simulink model "MPPT_solar_sim"  (R2019b)
settings: Solver=VariableStepAuto  StartTime=0.0  StopTime=10  RelTol=1e-3
undefined symbols (not defined in the file or in its folder): sigbuilder_block
libraries: powerlib x10, re_lib x1, powerlib_meascontrol x1
settings Model: Creator=root  LastModifiedBy=root

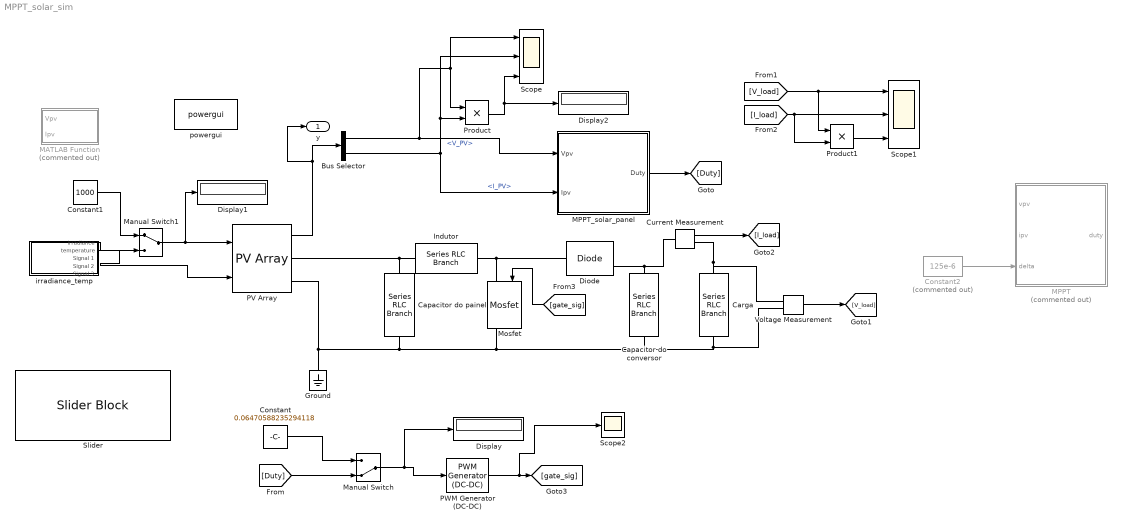
== system MPPT_solar_sim ==
  Bus Selector : BusSelector  OutputSignals=V_PV,I_PV
  Capacitor do conversor : powerlib/Elements/Series RLC Branch  LConnTagsString=__new0  RConnTagsString=__new0  BranchType=C  Resistance=1e-4  Inductance=1e-3  SetiL0=off  InitialCurrent=0  Capacitance=500e-6  Setx0=off  InitialVoltage=0  Measurements=None
      settings: SourceProductName=Simscape Electrical
  Capacitor do painel : powerlib/Elements/Series RLC Branch  LConnTagsString=__new0  RConnTagsString=__new0  BranchType=C  Resistance=1e-4  Inductance=1e-3  SetiL0=off  InitialCurrent=0  Capacitance=100e-6  Setx0=off  InitialVoltage=0  Measurements=None
      settings: SourceProductName=Simscape Electrical
  "Carga " : powerlib/Elements/Series RLC Branch  LConnTagsString=__new0  RConnTagsString=__new0  BranchType=R  Resistance=10  Inductance=1e-3  SetiL0=off  InitialCurrent=0  Capacitance=20e-6  Setx0=off  InitialVoltage=0  Measurements=None
      settings: SourceProductName=Simscape Electrical
  Constant : Constant  Value=0.06470588235294118
  Constant1 : Constant  Value=1000
  Constant2 : Constant  Commented=on  Value=125e-6
  Current Measurement : powerlib/Measurements/Current Measurement  PhasorSimulation=off  OutputType=Complex  PSBequivalent=0
      settings: SourceProductName=Simscape Electrical
  Diode : powerlib/Power Electronics/Diode  Ron=0.001  Lon=0  Vf=0.8  IC=0  UseSnubber=0  Rs=500  Cs=250e-9  Measurements=on
      settings: SourceProductName=Simscape Electrical
  Display : Display
  Display1 : Display
  Display2 : Display
  Ground : powerlib/Elements/Ground  LConnTagsString=a
      settings: SourceProductName=Simscape Electrical
  Indutor : powerlib/Elements/Series RLC Branch  LConnTagsString=__new0  RConnTagsString=__new0  BranchType=L  Resistance=1e-4  Inductance=235e-6  SetiL0=off  InitialCurrent=0  Capacitance=100e-6  Setx0=off  InitialVoltage=0  Measurements=None
      settings: SourceProductName=Simscape Electrical
  MATLAB Function : MATLAB Function  Commented=on  TreatAsAtomicUnit=on
  MPPT : MATLAB Function  Commented=on  TreatAsAtomicUnit=on
  "MPPT_solar_panel " : MATLAB Function  TreatAsAtomicUnit=on
  Manual Switch : ManualSwitch  CurrentSetting=0
  Manual Switch1 : ManualSwitch
  Mosfet : powerlib/Power Electronics/Mosfet  Ron=0.1  Lon=0  Rd=0.01  Vfd=0  IC=0  Rs=1e5  Cs=inf  Measurements=on
      settings: SourceProductName=Simscape Electrical
  PV Array : re_lib/Solar/PV Array  Npar=1  Nser=1  PlotType=one module @ 25 deg.C & specified irradiances  S_vec="[ 1000  800  600 400 200]"  Temp_C_vec="[ 45 25  ]"  ModuleName=User-defined  PlotWhenSelected=off  Pm=400.488  Ncell=60  Voc=48.70  Isc=10.79  Vm=40.70  Im=9.84  beta_Voc_pc=-0.289  alpha_Isc_pc=0.051  beta_Voc=-0.14074  alpha_Isc=0.0055029  IL=10.8217  I0=2.2788e-11  nI=1.1776  Rsh=79.7466  Rs=0.23394  BAL=on  Tc=1e-6  Tfilter=1e-3
      settings: SourceProductName=Simscape Electrical
  PWM Generator (DC-DC) : powerlib_meascontrol/Pulse & Signal Generators/PWM Generator (DC-DC)  Fsw=30e3  Ts=0
      settings: SourceProductName=Simscape Electrical
  Product : Product
  Product1 : Product
  Scope : Scope  NumInputPorts=3
  Scope1 : Scope  NumInputPorts=3
  Scope2 : Scope
  Slider : SliderBlock  ScaleMax=1
  Voltage Measurement : powerlib/Measurements/Voltage Measurement  PhasorSimulation=off  OutputType=Complex  PSBequivalent=0
      settings: SourceProductName=Simscape Electrical
  irradiance_temp : Subsystem  Tag=STV Subsys  LoadFcn=sigbuilder_block('load');  StartFcn=sigbuilder_block('start');  StopFcn=sigbuilder_block('stop');  ClipboardFcn=sigbuilder_block('clipboard');  mask(Sigbuilder block){tuvar=[0:10]}
      mask help: Simulink:masks:SigbuilderBlock_MD
      mask init:
      | if ~strcmp(get_param(bdroot(gcbh),'SimulationStatus'),'stopped') tuvar = sigbuilder_block('maskInit'); end
      settings: CopyFcn=sigbuilder_block('copy');  DeleteFcn=sigbuilder_block('delete');  ModelCloseFcn=sigbuilder_block('modelClose');  PreSaveFcn=sigbuilder_block('preSave');  PauseFcn=sigbuilder_block('pause');  ContinueFcn=sigbuilder_block('continue');  NameChangeFcn=sigbuilder_block('namechange');  OpenFcn=sigbuilder_block('open',[0 0 1868.11 814.378 ]);  CloseFcn=sigbuilder_block('close');
      mask Display: plot(0, 0, 100, 100,[2, 2, 32, 32, 2], [68, 8, 8, 68, 68],[32, 2], [38, 38], [32, 19, 2],[53, 60, 44], [32, 17, 17, 2],[16, 16, 31, 31]);txt = getActiveGroup(gcbh);text(2, 100, txt,'verticalAlignment', 'top');
  powergui : powerlib/powergui  Priority=1  SimulationMode=Discrete  SampleTime=1e-6  frequency=60  Iterations=50  frequencyindice=0  Pbase=100e6  ErrMax=1e-4  UnitsV=kV  UnitsW=MW  buscounter=0  FunctionMessages=off  echomessages=off  EnableUseOfTLC=off  CurrentSourceSwitches=off  DisableSnubberDevices=off  DisableRonSwitches=off  DisableVfSwitches=off  DisplayEquations=off  AutomaticDiscreteSolvers=off  SolverType=Tustin/Backward Euler (TBE)  Interpol=off  ExternalGateDelay=off  methode=off  Ts=100  x0status=blocks  SPID=on  SwTol=0  HookPort=off  NonlinearTolerance=1e-4  nMaxIteration=100  ContinueOnMaxIteration=off  RestoreLinks=warning  ResistiveCurrentMeasurement=off  Frange=[0:2:500]  Ylog=off  Xlog=on  ShowGrid=off  save=off  variable=ZData  structure=0  ZoomFFT=off  StartTime=0.0  cycles=1  DisplayStyle=1  fundamental=60  FreqAxis=off  MaxFrequency=1000  frequencyindicesteady=1  RmsSteady=1  display=off
      settings: SourceProductName=Simscape Electrical
  " y" : Outport
  wires:
  Bus Selector/1 -> "MPPT_solar_panel "/1(Vpv), Product/1, Scope/1  "<V_PV>"
  Bus Selector/2 -> "MPPT_solar_panel "/2(Ipv), Scope/2, Product/2  "<I_PV>"
  PV Array/1 -> Bus Selector/1, " y"/1
  irradiance_temp/2(temperature) -> PV Array/2
  Voltage Measurement/1 -> [V_load]
  Current Measurement/1 -> [I_load]
  [V_load] -> Product1/1, Scope1/1
  [I_load] -> Scope1/2, Product1/2
  PWM Generator (DC-DC)/1 -> Scope2/1, [gate_sig]
  Product/1 -> Display2/1, Scope/3
  [Duty] -> Manual Switch/2
  Manual Switch/1 -> Display/1, PWM Generator (DC-DC)/1
  Constant/1 -> Manual Switch/1
  Product1/1 -> Scope1/3
  irradiance_temp/1(irradiance) -> Manual Switch1/2
  Manual Switch1/1 -> Display1/1, PV Array/1
  Constant1/1 -> Manual Switch1/1
  [gate_sig] -> Mosfet/1
  Constant2/1 -> MPPT/3(delta)
  "MPPT_solar_panel "/1(Duty) -> [Duty]
  connections:
  PV Array/RConn2 -- Mosfet/RConn1 -- Voltage Measurement/LConn2 -- "Carga "/RConn1 -- Capacitor do conversor/RConn1 -- Capacitor do painel/RConn1 -- Ground/LConn1
  "Carga "/LConn1 -- Voltage Measurement/LConn1 -- Current Measurement/RConn1
  Current Measurement/LConn1 -- Diode/RConn1 -- Capacitor do conversor/LConn1
  Capacitor do painel/LConn1 -- PV Array/RConn1 -- Indutor/RConn1
  Mosfet/LConn1 -- Diode/LConn1 -- Indutor/LConn1

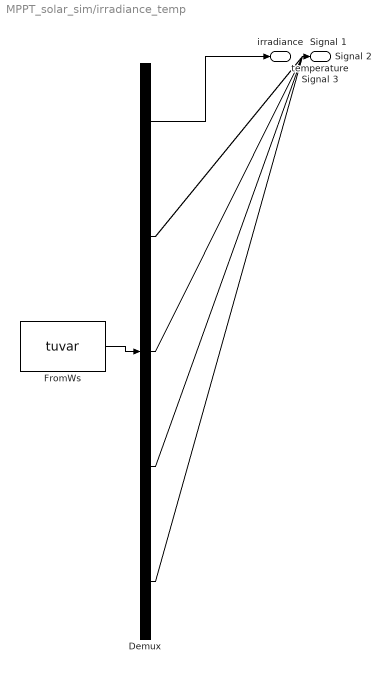
== system MPPT_solar_sim/irradiance_temp ==
  Demux : Demux  Tag=STV Demux  Outputs=5
  FromWs : FromWorkspace  Tag=STV FromWs  VariableName=tuvar  SampleTime=0
      SigBuilderData=|
      | common.afterFinalStr = 'Extrapolate'
      | common.sampleTime = 0
      | dataSet.timeRange = [0 10]
      | dataSet.name = 'Group 1'
      | sbobj.Groups.Name = 'Group 1'
      | sbobj.Groups.Signals(1).Name = 'irradiance'
      | sbobj.Groups.Signals(1).XData = [0 1 1.001 2 2.001 3 10]
      | sbobj.Groups.Signals(1).YData = [200 200 400 400 600 1000 1000]
      | sbobj.Groups.Signals(2).Name = 'temperature'
      | sbobj.Groups.Signals(2).XData = [0 5 10]
      | sbobj.Groups.Signals(2).YData = [25 25 25]
      | sbobj.Groups.Signals(3).Name = 'Signal 1'
      | sbobj.Groups.Signals(3).XData = [0 4 4 6 6 10]
      | sbobj.Groups.Signals(3).YData = [0 0 1 1 0 0]
      | sbobj.Groups.Signals(4).Name = 'Signal 2'
      | sbobj.Groups.Signals(4).XData = [0 2 4 6 8 10]
      | sbobj.Groups.Signals(4).YData = [200 400 600 800 900 999]
      | sbobj.Groups.Signals(5).Name = 'Signal 3'
      | sbobj.Groups.Signals(5).XData = [0 1 1 2 2 3 3 4 4 5 5 6 6 7 7 8 8 9 9 10]
      | sbobj.Groups.Signals(5).YData = [0 2 0.12 1.86 0 2 0 2 0 2 0 2 0 2 0 2 0 2 0 2]
  irradiance : Outport  Tag=STV Outport
  temperature : Outport  Tag=STV Outport  Port=2
  Signal 1 : Outport  Tag=STV Outport  Port=3
  Signal 2 : Outport  Tag=STV Outport  Port=4
  Signal 3 : Outport  Tag=STV Outport  Port=5
  wires:
  Demux/1 -> irradiance/1
  FromWs/1 -> Demux/1
  Demux/2 -> temperature/1
  Demux/3 -> Signal 1/1
  Demux/4 -> Signal 2/1
  Demux/5 -> Signal 3/1

== matlab function MPPT_solar_sim/MPPT_solar_panel  ==
  data: Vpv input; Duty output; Ipv input
% Codigo para algoritmo MPPT pertubation and observation
% para o painel fotovoltaico.

function Duty = MPPT_solar_panel(Vpv, Ipv)


    %% Declaramos as variaveis do tipo persistent de forma que os valores 
    % fiquem armazenados mesmo com o término da função
    
    persistent Vpv_old Ppv_old Duty_old
    
    % Inicializacao das variaveis
    if isempty(Duty_old)
       Duty_old = 0.5;
       Ppv_old = 0;
       Vpv_old = 0;
    end
    
    Duty_var = 125e-6;           % Delta de variacao a cada iteracao
    
    
    % Calculo do valor de potencia
    
    Ppv = Vpv * Ipv;
    
    %% Inicializacao da comparacao
    
    if ((Ppv - Ppv_old) ~= 0)
       if ((Ppv - Ppv_old) < 0) 
            if ((Vpv - Vpv_old) < 0)
                Duty = Duty_old - Duty_var;
            else 
                Duty = Duty_old + Duty_var;
            end
       else 
           if ((Vpv - Vpv_old) < 0)
                Duty = Duty_old + Duty_var;
           else 
               Duty = Duty_old - Duty_var;
           end
       end
    else 
        
        Duty = Duty_old;
        
    end
    
    if (Duty > 1)
        Duty = 1.0;
    elseif Duty < 0
        Duty = 0.0;
    end 
    
    Ppv_old = Ppv;
    Vpv_old = Vpv;
    Duty_old = Duty;    
end

== matlab function MPPT_solar_sim/MATLAB Function ==
  data: Vpv input; Ipv input
% Função para plotagem do grafico de tensao por potencia

function fcn(Vpv, Ipv)

    % Primeiro, obtemos a potencia
    
    Ppv = Vpv * Ipv;
    
    % Iniciamos a plotagem do grafico
    % Vamos defnir a voltagem variando de zero a 40
    figure(1)
    plot(Vpv, Ppv, 'r')
    xlim([0 40])
    


end

== matlab function MPPT_solar_sim/MPPT ==
  data: vpv input; duty output; ipv input; delta input
function duty = MPPT_algorithm(vpv,ipv,delta)
% I used the MPPT algorithm in the MATLAB examples
% I only modify somethings.
duty_init = 0.1;
% min and max value are used to limit duty between
% 0 and 0.85
duty_min=0;
duty_max=0.85;

persistent Vold Pold duty_old;
% persistent variable type can be store the data
% we need the old data by obtain difference
% between old and new value
if isempty(Vold)
    Vold=0;
    Pold=0;
    duty_old=duty_init;
end
P= vpv*ipv; % power
dV= vpv - Vold; % difference between old and new voltage
dP= P - Pold;% difference between old and new power

% the algorithm in below search the dP/dV=0
% if the derivative equal to zero
% duty will not change
% if old and new power not equal
% &
% pv voltage bigger than 30V
% the algorithm will works
if dP ~= 0
    if dP < 0
        if dV < 0
            duty = duty_old - delta;
        else
            duty = duty_old + delta;
        end
    else
        if dV < 0
            duty = duty_old + delta;
        else
            duty = duty_old - delta;
        end
    end
else
    duty = duty_old;
end

%the below if limits the duty between min and max
if duty >= duty_max
    duty=duty_max;
elseif duty<duty_min
    duty=duty_min;
end

% stored data
duty_old=duty;
Vold=vpv;
Pold=P;
